simulink model "sim_part2"  (R2020a)
settings: Solver=VariableStepAuto  StartTime=0.0  StopTime=10.0  RelTol=1e-3
values from neighbouring files (symbols this model uses):
  gov = 0.5    [part1.m]    (also in part2.m; part3.m)
  i_b_m = 0.025    [part1.m]    (also in part2.m; part3.m; stability_plot.m)
  i_cb = 0.1    [part1.m]    (also in part2.m; part3.m; stability_plot.m)
  i_f_m = 0.05    [part1.m]    (also in part2.m; part3.m; stability_plot.m)
  K_0 = 0.08    [part1.m]    (also in part2.m; part3.m; stability_plot.m)
  K_p = 15    [part1.m]    (also in part2.m; part3.m; stability_plot.m)
  lambda = 0.002    [part1.m]    (also in part2.m; part3.m; stability_plot.m)
  lambda_f = 0.005    [part1.m]    (also in part2.m; part3.m; stability_plot.m)
  loss_eq = 2    [part1.m]    (also in part2.m; part3.m; stability_plot.m)
  R = 1    [part1.m]    (also in part2.m; part3.m; stability_plot.m)
  r_f = 0.1    [part1.m]    (also in part2.m; part3.m; stability_plot.m)
  rate = 0.1    [part1.m]    (also in part2.m; part3.m)
  s_k = 0.2    [part1.m]    (also in part2.m; part3.m)
  sigma = 0.28    [part1.m]    (also in part2.m; part3.m)
  T_f = 0.5    [part1.m]    (also in part2.m; part3.m; stability_plot.m)
  T_g = 1    [part1.m]    (also in part2.m; part3.m; stability_plot.m)
  T_h = 0.1    [part1.m]    (also in part2.m; part3.m; stability_plot.m)
  T_i = 8    [part1.m]    (also in part2.m; part3.m; stability_plot.m)
  T_k = 0.1    [part1.m]    (also in part2.m; part3.m; stability_plot.m)
  tx = 0.3    [part1.m]    (also in part2.m; part3.m)
settings Model: Creator=erlended  LastModifiedBy=erlended

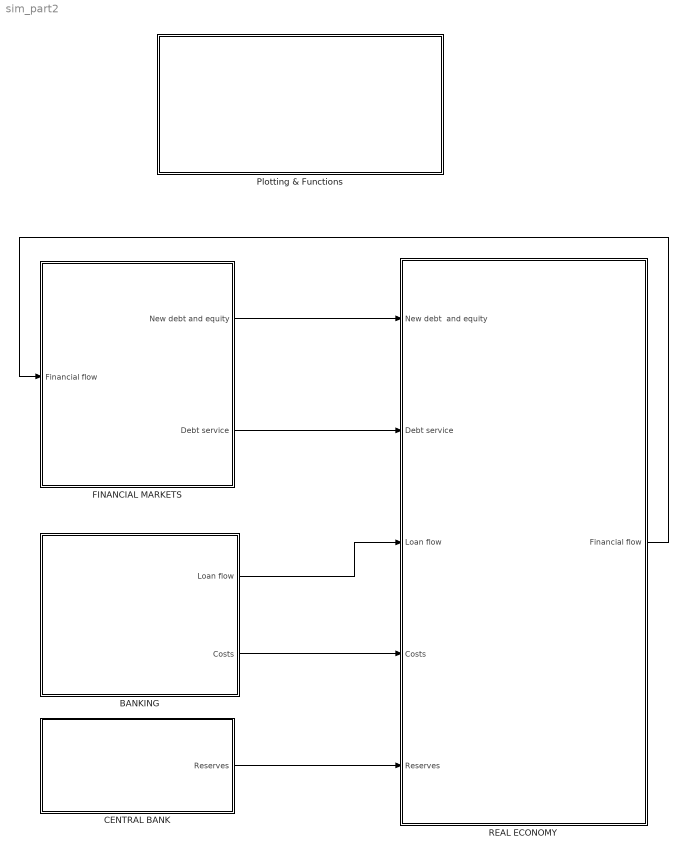
== system sim_part2 ==
  BANKING : Subsystem
  CENTRAL BANK : Subsystem
  FINANCIAL MARKETS : Subsystem
  Plotting & Functions : Subsystem
  REAL ECONOMY : Subsystem
  wires:
  BANKING/1(Loan flow) -> REAL ECONOMY/3(Loan flow)
  BANKING/2(Costs) -> REAL ECONOMY/4(Costs)
  CENTRAL BANK/1(Reserves) -> REAL ECONOMY/5(Reserves)
  FINANCIAL MARKETS/1(New debt and equity) -> REAL ECONOMY/1(New debt  and equity)
  FINANCIAL MARKETS/2(Debt service) -> REAL ECONOMY/2(Debt service)
  REAL ECONOMY/1(Financial flow) -> FINANCIAL MARKETS/1(Financial flow)

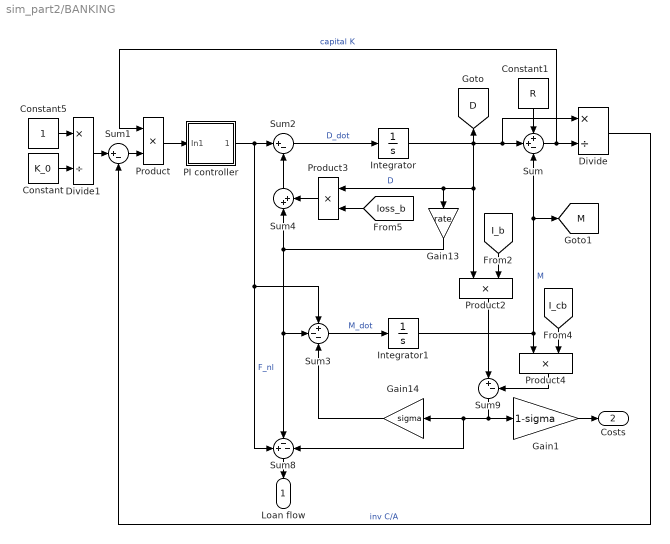
== system sim_part2/BANKING ==
  Constant : Constant  Value=K_0
  Constant1 : Constant  Value=R
  Constant5 : Constant
  Divide : Product  Inputs=*/
  Divide1 : Product  Inputs=*/
  Gain1 : Gain  Gain=1-sigma
  Gain13 : Gain  Gain=rate
  Gain14 : Gain  Gain=sigma
  Integrator : Integrator
  Integrator1 : Integrator
  PI controller : Subsystem
  Product{,2..4} (4 alike) : Product
  Sum : Sum  Inputs=++-
  Sum1 : Sum  Inputs=|+-
  Sum2 : Sum  Inputs=|+-
  Sum3 : Sum  Inputs=+--
  Sum4 : Sum  Inputs=|++
  Sum8 : Sum  Inputs=+--
  Sum9 : Sum  Inputs=|+-
  Loan flow : Outport
  Costs : Outport  Port=2
  tag scope: D=global, M=global
  wires:
  Integrator/1 -> [D], Product3/1, Gain13/1, Product2/1, Sum/2, Divide/1  "D"
  Sum8/1 -> Loan flow/1
  Integrator1/1 -> Product4/1, [M], Sum/3  "M"
  Sum/1 -> Divide/2, Product/1  "capital K"
  Sum4/1 -> Sum2/2
  Gain13/1 -> Sum8/2, Sum3/2, Sum4/1
  Sum9/1 -> Gain14/1, Sum8/3, Gain1/1
  Sum2/1 -> Integrator/1  "D_dot"
  Constant1/1 -> Sum/1
  Divide/1 -> Sum1/2  "inv C/A"
  Sum1/1 -> Product/2
  Sum3/1 -> Integrator1/1  "M_dot"
  Product2/1 -> Sum9/1
  Product4/1 -> Sum9/2
  Constant5/1 -> Divide1/1
  Divide1/1 -> Sum1/1
  Gain14/1 -> Sum3/3
  Gain1/1 -> Costs/1
  Constant/1 -> Divide1/2
  [I_b] -> Product2/2
  [I_cb] -> Product4/2
  [loss_b] -> Product3/2
  Product3/1 -> Sum4/2
  PI controller/1(Out1) -> Sum2/1, Sum8/1, Sum3/1  "F_nl"
  Product/1 -> PI controller/1(In1)

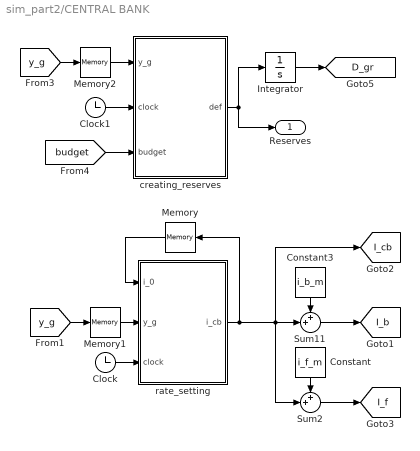
== system sim_part2/CENTRAL BANK ==
  Clock : Clock
  Clock1 : Clock
  Constant : Constant  Value=i_f_m
  Constant3 : Constant  Value=i_b_m
  Integrator : Integrator
  Memory : Memory  InitialCondition=i_cb
  Memory1 : Memory
  Memory2 : Memory
  Sum11 : Sum  Inputs=++|
  Sum2 : Sum  Inputs=++|
  creating_reserves : MATLAB Function  TreatAsAtomicUnit=on
  rate_setting : MATLAB Function  TreatAsAtomicUnit=on
  Reserves : Outport
  tag scope: D_gr=global, I_b=global, I_cb=global, I_f=global
  wires:
  Constant/1 -> Sum2/1
  rate_setting/1(i_cb) -> Memory/1, [I_cb], Sum11/2, Sum2/2
  Constant3/1 -> Sum11/1
  Sum11/1 -> [I_b]
  [y_g] -> Memory1/1
  Memory/1 -> rate_setting/1(i_0)
  Clock/1 -> rate_setting/3(clock)
  Memory1/1 -> rate_setting/2(y_g)
  [budget] -> creating_reserves/3(budget)
  Integrator/1 -> [D_gr]
  creating_reserves/1(def) -> Reserves/1, Integrator/1
  Clock1/1 -> creating_reserves/2(clock)
  [y_g] -> Memory2/1
  Memory2/1 -> creating_reserves/1(y_g)
  Sum2/1 -> [I_f]

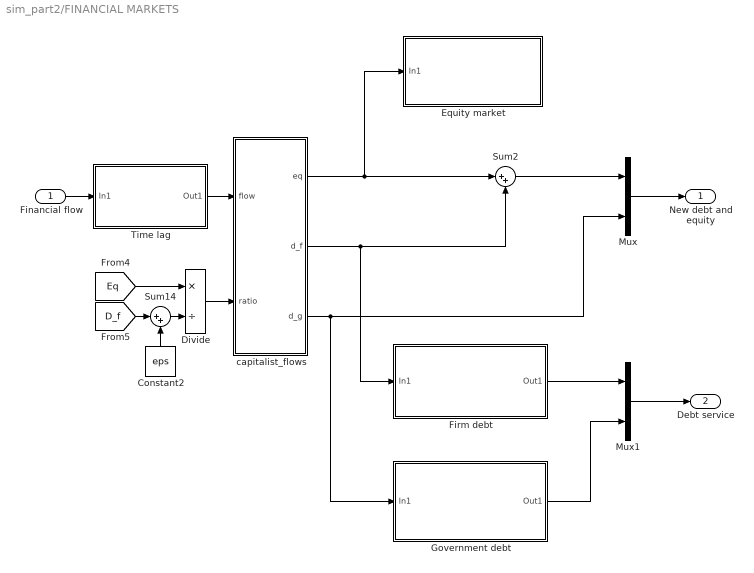
== system sim_part2/FINANCIAL MARKETS ==
  Financial flow : Inport
  Constant2 : Constant  Value=eps
  Divide : Product  Inputs=*/
  Equity market : Subsystem
  Firm debt : Subsystem
  Government debt : Subsystem
  Mux : Mux  Inputs=2
  Mux1 : Mux  Inputs=2
  Sum14 : Sum  Inputs=|++
  Sum2 : Sum  Inputs=|++
  "Time lag " : Subsystem
  capitalist_flows : MATLAB Function  TreatAsAtomicUnit=on
  New debt and equity : Outport
  Debt service : Outport  Port=2
  wires:
  Government debt/1(Out1) -> Mux1/2
  capitalist_flows/2(d_f) -> Sum2/2, Firm debt/1(In1)
  [Eq] -> Divide/1
  Sum2/1 -> Mux/1
  [D_f] -> Sum14/1
  capitalist_flows/3(d_g) -> Mux/2, Government debt/1(In1)
  Divide/1 -> capitalist_flows/2(ratio)
  "Time lag "/1(Out1) -> capitalist_flows/1(flow)
  Constant2/1 -> Sum14/2
  Sum14/1 -> Divide/2
  capitalist_flows/1(eq) -> Sum2/1, Equity market/1(In1)
  Firm debt/1(Out1) -> Mux1/1
  Financial flow/1 -> "Time lag "/1(In1)
  Mux/1 -> New debt and equity/1
  Mux1/1 -> Debt service/1

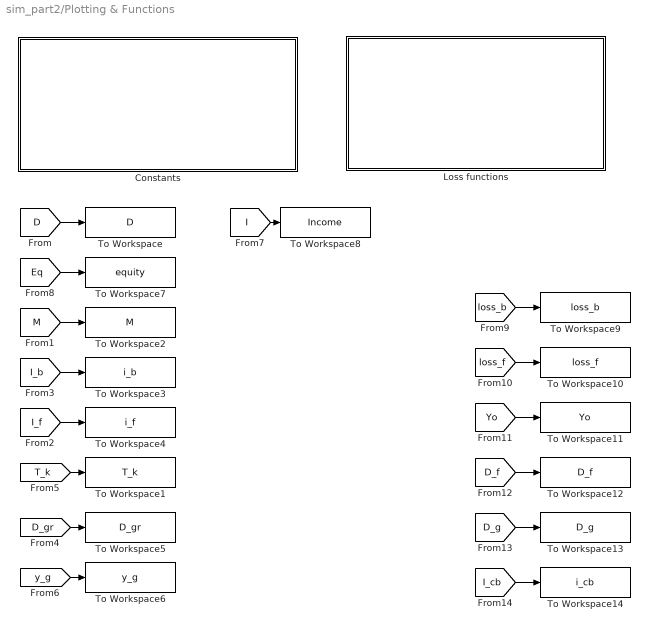
== system sim_part2/Plotting & Functions ==
  Constants : Subsystem
  Loss functions : Subsystem
  To Workspace : ToWorkspace  VariableName=D  SaveFormat=Timeseries  SampleTime=-1
  To Workspace1 : ToWorkspace  VariableName=T_k  SaveFormat=Timeseries  SampleTime=-1
  To Workspace10 : ToWorkspace  VariableName=loss_f  SaveFormat=Timeseries  SampleTime=-1
  To Workspace11 : ToWorkspace  VariableName=Yo  SaveFormat=Timeseries  SampleTime=-1
  To Workspace12 : ToWorkspace  VariableName=D_f  SaveFormat=Timeseries  SampleTime=-1
  To Workspace13 : ToWorkspace  VariableName=D_g  SaveFormat=Timeseries  SampleTime=-1
  To Workspace14 : ToWorkspace  VariableName=i_cb  SaveFormat=Timeseries  SampleTime=-1
  To Workspace2 : ToWorkspace  VariableName=M  SaveFormat=Timeseries  SampleTime=-1
  To Workspace3 : ToWorkspace  VariableName=i_b  SaveFormat=Timeseries  SampleTime=-1
  To Workspace4 : ToWorkspace  VariableName=i_f  SaveFormat=Timeseries  SampleTime=-1
  To Workspace5 : ToWorkspace  VariableName=D_gr  SaveFormat=Timeseries  SampleTime=-1
  To Workspace6 : ToWorkspace  VariableName=y_g  SaveFormat=Timeseries  SampleTime=-1
  To Workspace7 : ToWorkspace  VariableName=equity  SaveFormat=Timeseries  SampleTime=-1
  To Workspace8 : ToWorkspace  VariableName=Income  SaveFormat=Timeseries  SampleTime=-1
  To Workspace9 : ToWorkspace  VariableName=loss_b  SaveFormat=Timeseries  SampleTime=-1
  wires:
  [D] -> To Workspace/1
  [Eq] -> To Workspace7/1
  [M] -> To Workspace2/1
  [I_b] -> To Workspace3/1
  [I_f] -> To Workspace4/1
  [D_gr] -> To Workspace5/1
  [T_k] -> To Workspace1/1
  [y_g] -> To Workspace6/1
  [I] -> To Workspace8/1
  [loss_b] -> To Workspace9/1
  [loss_f] -> To Workspace10/1
  [Yo] -> To Workspace11/1
  [D_f] -> To Workspace12/1
  [D_g] -> To Workspace13/1
  [I_cb] -> To Workspace14/1

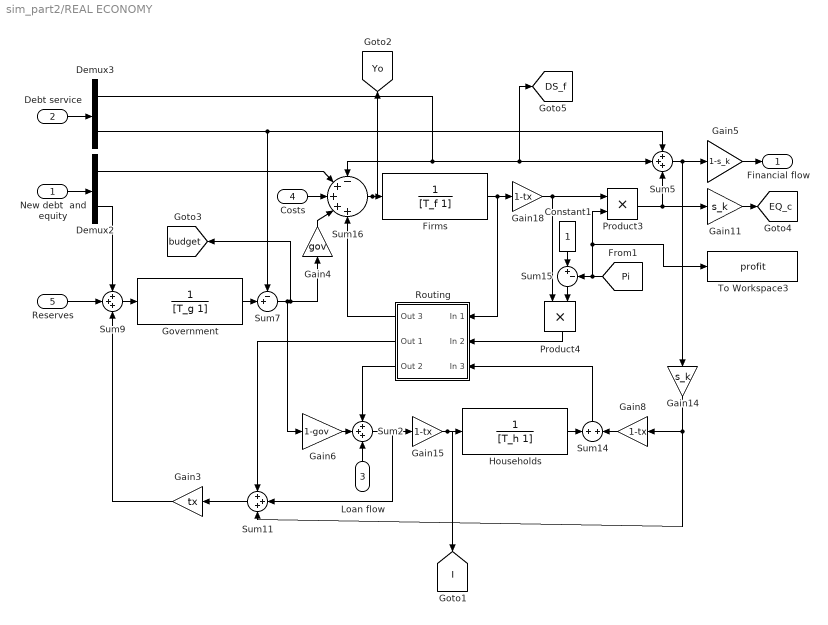
== system sim_part2/REAL ECONOMY ==
  New debt  and equity : Inport
  Debt service : Inport  Port=2
  Loan flow : Inport  Port=3
  Costs : Inport  Port=4
  Reserves : Inport  Port=5
  Constant1 : Constant
  Demux2 : Demux  Outputs=2
  Demux3 : Demux  Outputs=2
  Firms : TransferFcn  Denominator=[T_f 1]
  Gain11 : Gain  Gain=s_k
  Gain14 : Gain  Gain=s_k
  Gain15 : Gain  Gain=1-tx
  Gain18 : Gain  Gain=1-tx
  Gain3 : Gain  Gain=tx
  Gain4 : Gain  Gain=gov
  Gain5 : Gain  Gain=1-s_k
  Gain6 : Gain  Gain=1-gov
  Gain8 : Gain  Gain=1-tx
  Government : TransferFcn  Denominator=[T_g 1]
  Households : TransferFcn  Denominator=[T_h 1]
  Product3 : Product
  Product4 : Product
  Routing : Subsystem
  Sum{2,5,9,11} (4 alike) : Sum  Inputs=+++
  Sum14 : Sum  Inputs=+|+
  Sum15 : Sum  Inputs=|+-
  Sum16 : Sum  Inputs=-++++
  Sum7 : Sum  Inputs=-+|
  To Workspace3 : ToWorkspace  VariableName=profit  SaveFormat=Timeseries  SampleTime=-1
  Financial flow : Outport
  tag scope: DS_f=global, EQ_c=global, I=global, Yo=global, budget=global
  wires:
  Reserves/1 -> Sum9/2
  Gain11/1 -> [EQ_c]
  Gain4/1 -> Sum16/4
  Routing/1(Out 3) -> Sum16/5
  Sum16/1 -> [Yo], Firms/1
  Product4/1 -> Routing/2(In 2)
  Constant1/1 -> Sum15/1
  Sum2/1 -> Gain15/1, Sum11/2
  Sum9/1 -> Government/1
  Loan flow/1 -> Sum2/3
  Gain5/1 -> Financial flow/1
  Costs/1 -> Sum16/3
  Routing/2(Out 1) -> Sum11/1
  Firms/1 -> Routing/1(In 1), Gain18/1
  Sum14/1 -> Routing/3(In 3)
  Debt service/1 -> Demux3/1
  Gain18/1 -> Product4/1, Product3/1
  Gain8/1 -> Sum14/2
  Demux3/2 -> Sum5/1, Sum7/1
  Gain6/1 -> Sum2/2
  Routing/3(Out 2) -> Sum2/1
  Gain15/1 -> [I], Households/1
  Gain14/1 -> Sum11/3, Gain8/1
  [Pi] -> Sum15/2, To Workspace3/1, Product3/2
  Households/1 -> Sum14/1
  Sum5/1 -> Gain5/1, Gain14/1
  Demux3/1 -> [DS_f], Sum5/2, Sum16/1
  Sum15/1 -> Product4/2
  Product3/1 -> Sum5/3, Gain11/1
  Demux2/2 -> Sum9/1
  Sum7/1 -> Gain4/1, [budget], Gain6/1
  New debt  and equity/1 -> Demux2/1
  Government/1 -> Sum7/2
  Gain3/1 -> Sum9/3
  Sum11/1 -> Gain3/1
  Demux2/1 -> Sum16/2

== system sim_part2/BANKING/PI controller ==
  In1 : Inport
  Gain3 : Gain  Gain=K_p
  Saturation : Saturate  UpperLimit=1000  LowerLimit=0
  Transfer Fcn : TransferFcn  Numerator=[T_i 1]  Denominator=[T_i 0]
  Out1 : Outport
  wires:
  Gain3/1 -> Transfer Fcn/1
  Transfer Fcn/1 -> Saturation/1
  In1/1 -> Gain3/1
  Saturation/1 -> Out1/1

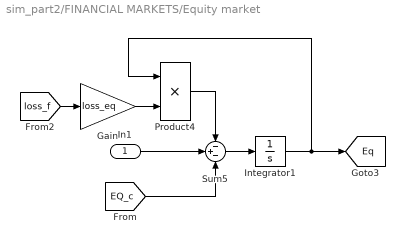
== system sim_part2/FINANCIAL MARKETS/Equity market ==
  In1 : Inport
  Gain : Gain  Gain=loss_eq
  Integrator1 : Integrator
  Product4 : Product
  Sum5 : Sum  Inputs=-+-
  tag scope: Eq=global
  wires:
  Sum5/1 -> Integrator1/1
  [EQ_c] -> Sum5/3
  Product4/1 -> Sum5/1
  In1/1 -> Sum5/2
  Integrator1/1 -> [Eq], Product4/1
  [loss_f] -> Gain/1
  Gain/1 -> Product4/2

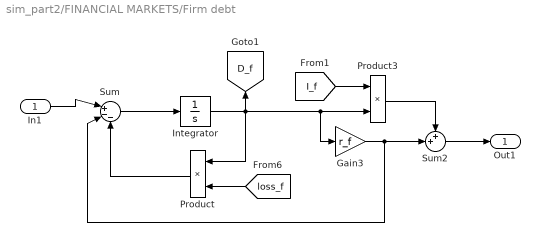
== system sim_part2/FINANCIAL MARKETS/Firm debt ==
  In1 : Inport
  Gain3 : Gain  Gain=r_f
  Integrator : Integrator
  Product : Product
  Product3 : Product
  Sum : Sum  Inputs=|+--
  Sum2 : Sum  Inputs=++|
  Out1 : Outport
  tag scope: D_f=global
  wires:
  In1/1 -> Sum/1
  Sum2/1 -> Out1/1
  [loss_f] -> Product/2
  [I_f] -> Product3/1
  Sum/1 -> Integrator/1
  Integrator/1 -> Product/1, Product3/2, Gain3/1, [D_f]
  Product3/1 -> Sum2/1
  Product/1 -> Sum/3
  Gain3/1 -> Sum/2, Sum2/2

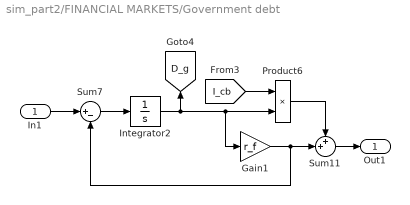
== system sim_part2/FINANCIAL MARKETS/Government debt ==
  In1 : Inport
  Gain1 : Gain  Gain=r_f
  Integrator2 : Integrator
  Product6 : Product
  Sum11 : Sum  Inputs=++|
  Sum7 : Sum  Inputs=|+-
  Out1 : Outport
  tag scope: D_g=global
  wires:
  Integrator2/1 -> [D_g], Product6/2, Gain1/1
  Sum7/1 -> Integrator2/1
  In1/1 -> Sum7/1
  [I_cb] -> Product6/1
  Gain1/1 -> Sum7/2, Sum11/2
  Product6/1 -> Sum11/1
  Sum11/1 -> Out1/1

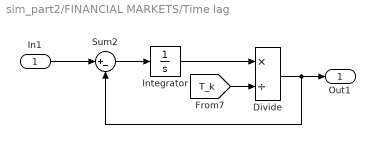
== system sim_part2/FINANCIAL MARKETS/Time lag  ==
  In1 : Inport
  Divide : Product  Inputs=*/
  Integrator : Integrator
  Sum2 : Sum  Inputs=|+-
  Out1 : Outport
  wires:
  In1/1 -> Sum2/1
  Sum2/1 -> Integrator/1
  Divide/1 -> Out1/1, Sum2/2
  Integrator/1 -> Divide/1
  [T_k] -> Divide/2

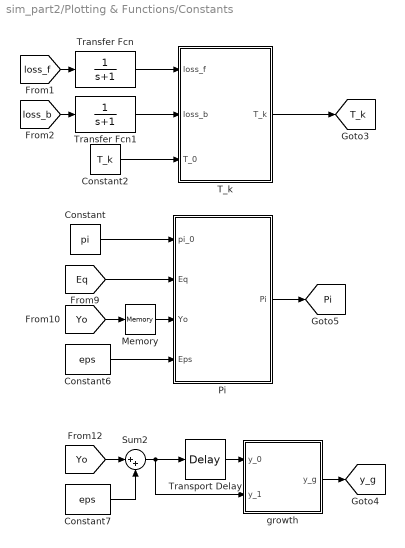
== system sim_part2/Plotting & Functions/Constants ==
  Constant : Constant  Value=pi
  Constant2 : Constant  Value=T_k
  Constant6 : Constant  Value=eps
  Constant7 : Constant  Value=eps
  Memory : Memory
  Pi : MATLAB Function  TreatAsAtomicUnit=on
  Sum2 : Sum  Inputs=|++
  T_k : MATLAB Function  TreatAsAtomicUnit=on
  Transfer Fcn : TransferFcn  Denominator=[1 1]
  Transfer Fcn1 : TransferFcn  Denominator=[1 1]
  Transport Delay : TransportDelay
  growth : MATLAB Function  TreatAsAtomicUnit=on
  tag scope: Pi=global, T_k=global, y_g=global
  wires:
  Pi/1(Pi) -> [Pi]
  T_k/1(T_k) -> [T_k]
  [Eq] -> Pi/2(Eq)
  Memory/1 -> Pi/3(Yo)
  Constant/1 -> Pi/1(pi_0)
  [Yo] -> Memory/1
  Constant2/1 -> T_k/3(T_0)
  Constant6/1 -> Pi/4(Eps)
  Transfer Fcn/1 -> T_k/1(loss_f)
  [loss_f] -> Transfer Fcn/1
  [loss_b] -> Transfer Fcn1/1
  Transfer Fcn1/1 -> T_k/2(loss_b)
  growth/1(y_g) -> [y_g]
  Sum2/1 -> Transport Delay/1, growth/2(y_1)
  Transport Delay/1 -> growth/1(y_0)
  Constant7/1 -> Sum2/2
  [Yo] -> Sum2/1

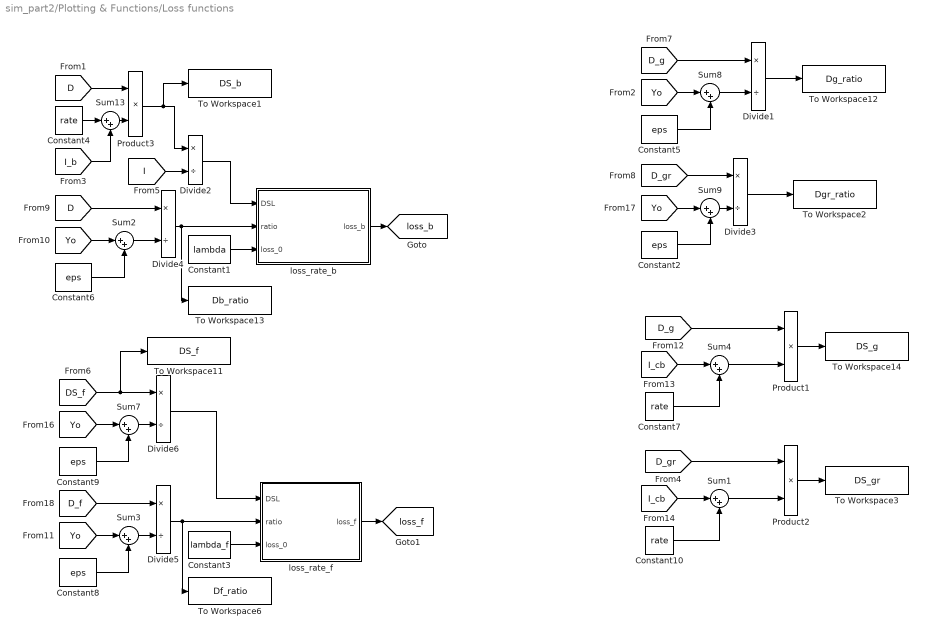
== system sim_part2/Plotting & Functions/Loss functions ==
  Constant1 : Constant  Value=lambda
  Constant10 : Constant  Value=rate
  Constant{2,5..6,8..9} (5 alike) : Constant  Value=eps
  Constant3 : Constant  Value=lambda_f
  Constant4 : Constant  Value=rate
  Constant7 : Constant  Value=rate
  Divide{1..6} (6 alike) : Product  Inputs=*/
  Product1 : Product
  Product2 : Product
  Product3 : Product
  Sum{1..4,7..9,13} (8 alike) : Sum  Inputs=|++
  To Workspace1 : ToWorkspace  VariableName=DS_b  SaveFormat=Timeseries  SampleTime=-1
  To Workspace11 : ToWorkspace  VariableName=DS_f  SaveFormat=Timeseries  SampleTime=-1
  To Workspace12 : ToWorkspace  VariableName=Dg_ratio  SaveFormat=Timeseries  SampleTime=-1
  To Workspace13 : ToWorkspace  VariableName=Db_ratio  SaveFormat=Timeseries  SampleTime=-1
  To Workspace14 : ToWorkspace  VariableName=DS_g  SaveFormat=Timeseries  SampleTime=-1
  To Workspace2 : ToWorkspace  VariableName=Dgr_ratio  SaveFormat=Timeseries  SampleTime=-1
  To Workspace3 : ToWorkspace  VariableName=DS_gr  SaveFormat=Timeseries  SampleTime=-1
  To Workspace6 : ToWorkspace  VariableName=Df_ratio  SaveFormat=Timeseries  SampleTime=-1
  loss_rate_b : MATLAB Function  TreatAsAtomicUnit=on
  loss_rate_f : MATLAB Function  TreatAsAtomicUnit=on
  tag scope: loss_b=global, loss_f=global
  wires:
  Constant1/1 -> loss_rate_b/3(loss_0)
  Constant4/1 -> Sum13/1
  Product3/1 -> To Workspace1/1, Divide2/1
  [D] -> Product3/1
  [I_b] -> Sum13/2
  [I] -> Divide2/2
  loss_rate_b/1(loss_b) -> [loss_b]
  Sum13/1 -> Product3/2
  Divide5/1 -> To Workspace6/1, loss_rate_f/2(ratio)
  loss_rate_f/1(loss_f) -> [loss_f]
  Constant3/1 -> loss_rate_f/3(loss_0)
  Divide1/1 -> To Workspace12/1
  Sum2/1 -> Divide4/2
  [D] -> Divide4/1
  Divide4/1 -> To Workspace13/1, loss_rate_b/2(ratio)
  Divide2/1 -> loss_rate_b/1(DSL)
  Divide6/1 -> loss_rate_f/1(DSL)
  Sum4/1 -> Product1/2
  Product1/1 -> To Workspace14/1
  [D_g] -> Product1/1
  [Yo] -> Sum2/1
  Constant6/1 -> Sum2/2
  Constant9/1 -> Sum7/2
  [Yo] -> Sum7/1
  Sum7/1 -> Divide6/2
  [DS_f] -> To Workspace11/1, Divide6/1
  Constant8/1 -> Sum3/2
  [Yo] -> Sum3/1
  Sum3/1 -> Divide5/2
  [D_f] -> Divide5/1
  Sum8/1 -> Divide1/2
  [Yo] -> Sum8/1
  Constant5/1 -> Sum8/2
  [D_g] -> Divide1/1
  [I_cb] -> Sum4/1
  Constant7/1 -> Sum4/2
  Constant2/1 -> Sum9/2
  Divide3/1 -> To Workspace2/1
  [Yo] -> Sum9/1
  Sum9/1 -> Divide3/2
  [D_gr] -> Divide3/1
  [D_gr] -> Product2/1
  Sum1/1 -> Product2/2
  [I_cb] -> Sum1/1
  Constant10/1 -> Sum1/2
  Product2/1 -> To Workspace3/1

== system sim_part2/REAL ECONOMY/Routing ==
  In 1 : Inport
  In 2 : Inport  Port=2
  In 3 : Inport  Port=3
  Out 3 : Outport
  Out 1 : Outport  Port=2
  Out 2 : Outport  Port=3
  wires:
  In 3/1 -> Out 3/1
  In 2/1 -> Out 2/1
  In 1/1 -> Out 1/1

== matlab function sim_part2/Plotting & Functions/Loss functions/loss_rate_b ==
  data: DSL input; ratio input; loss_b output; loss_0 input
function loss_b = fcn(DSL, ratio,loss_0)

loss_b = 0.0025*(ratio/1.6)^6+0.05*DSL^6+loss_0;

== matlab function sim_part2/FINANCIAL MARKETS/capitalist_flows ==
  data: flow input; eq output; d_f output; d_g output; ratio input
function [eq,d_f,d_g]= fcn(flow, ratio)
d_g = flow*0.2;

if ratio > 1
    eq = flow*(0.5 - 0.15*ratio);
    d_f = flow*(0.3 + 0.15*ratio);
else
    eq = flow*(0.5 + 0.15*ratio);
    d_f = flow*(0.3 - 0.15*ratio);
end

== matlab function sim_part2/Plotting & Functions/Loss functions/loss_rate_f ==
  data: DSL input; ratio input; loss_f output; loss_0 input
function loss_f = fcn(DSL, ratio,loss_0)

loss_f = 0.0015*(ratio)^4+(1.5*DSL)^4+loss_0;

== matlab function sim_part2/Plotting & Functions/Constants/T_k ==
  data: loss_f input; loss_b input; T_k output; T_0 input
function T_k = fcn(loss_f, loss_b, T_0)

%T_k = 0.55*(0.998+400*my)*T_0;
%T_k = 0.03*(ratio)^2+2*my+T_0;
T_k = 15*loss_f+60*loss_b+T_0;

== matlab function sim_part2/Plotting & Functions/Constants/Pi ==
  data: pi_0 input; Pi output; Eq input; Yo input; Eps input
function Pi = fcn(pi_0, Eq, Yo, Eps)

Pi = 0.05*Eq/(Yo+Eps)+pi_0;
if Pi > 0.6
    Pi = 0.6; 
end

== matlab function sim_part2/Plotting & Functions/Constants/growth ==
  data: y_0 input; y_g output; y_1 input
function y_g = fcn(y_0, y_1)

y_g = (y_1-y_0)/y_0;

== matlab function sim_part2/CENTRAL BANK/rate_setting ==
  data: i_0 input; y_g input; i_cb output; clock input
function i_cb = fcn(i_0, y_g, clock)

i_cb = i_0;

if y_g < 0.01 && clock > 5
    i_cb = i_0 - 0.005;
elseif y_g > 0.06 && clock > 5 
   i_cb = i_0 + 0.0025;
%elseif y_g > 0.04 && clock >= 50
%    i_cb = i_0 + 0.0025;
end

if i_cb <= 0
    i_cb = 0;
end

== matlab function sim_part2/CENTRAL BANK/creating_reserves ==
  data: y_g input; def output; clock input; budget input
function def = fcn(y_g, clock, budget)
def = 0;

if y_g < 0.06 && clock > 50 
    def = budget*0.05;
end
